simulink model "lookupTableDynamic_TestGen25"  (R2017b)
settings: Solver=FixedStepDiscrete  StartTime=0.0  StopTime=10.0  RelTol=1e-3
libraries: simulink x1
settings Model: Creator=ktrinh  LastModifiedBy=ktrinh
settings DebuggingCC: ParameterOverflowMsg=none

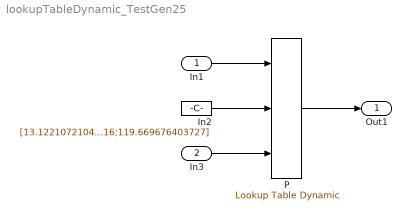
== system lookupTableDynamic_TestGen25 ==
  In1 : Inport  OutMin=11.1221  OutMax=121.6697  OutDataTypeStr=double  PortDimensions=1
  In3 : Inport  Port=2  PortDimensions=5
  In2 : Constant  Value=[13.1221072104475;26.2272618083899;37.5252735902115;41.4013593089016;119.669676403727]  OutDataTypeStr=double
  P : simulink/Lookup Tables/Lookup Table Dynamic  LookUpMeth=Use Input Below  OutDataType=fixdt('int32')  OutScaling=[]  OutputDataTypeScalingMode=Specify via dialog  OutDataTypeStr=int32  RndMeth=Round  DoSatur=on
      settings: SourceProductName=Simulink
  Out1 : Outport
  wires:
  In1/1 -> P/1
  In2/1 -> P/2
  In3/1 -> P/3
  P/1 -> Out1/1
